simulink model "TXsystem"  (R2024b)
settings: Solver=FixedStepAuto  StartTime=0.0  StopTime=inf  RelTol=1e-3
InitFcn:
  | symbolRate = 1e6;        % 1 MHz symbol rate
  | Ts = 1/symbolRate;       % Sample time per symbol
  | samplesPerSymbol = 8;    % Oversampling factor
  | Fs = symbolRate * samplesPerSymbol;  % 8 MHz sample rate
undefined symbols (not defined in the file or in its folder): ip, QAM, usb
libraries: plutoradiolib x1, commfilt2 x1, commdigbbndam3 x1
settings Model: Creator=J_mas  LastModifiedBy=J_mas

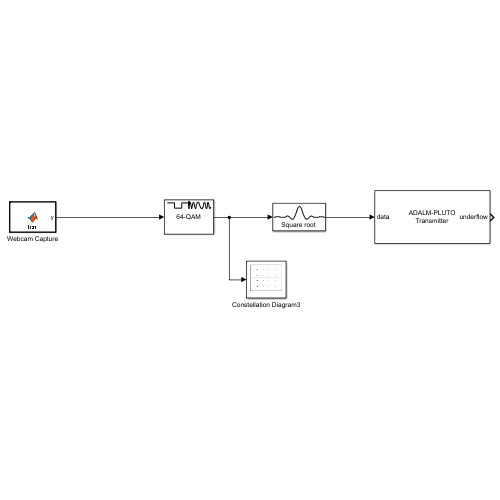
[thumbnail: Simulink's stored preview of the top-level diagram]
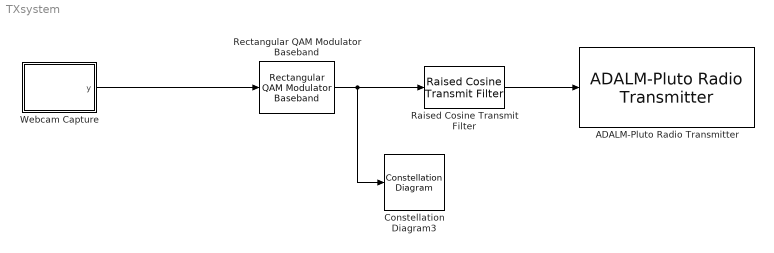
== system TXsystem ==
  ADALM-Pluto Radio Transmitter : plutoradiolib/ADALM-Pluto Radio Transmitter  RadioID=usb:0  uri=ip:10.0.0.200  CenterFrequencySource=Dialog  CenterFrequency=2.4e9  GainSource=Dialog  Gain=-10  ChannelMapping=1  BasebandSampleRate=1e6  UnderflowOutputPort=on  ShowAdvancedProperties=off  UseCustomFilter=off  filtPathRates=[737280000 11520000 3840000 1920000 960000 240000]  filtCoefficients=[-192 82 85 -215 228 -102 -110 290 -318 145 160 -426 471 -215 -238 633 -697 318 349 -923 1009 -457 -498 1309 -1423 640 693 -1812 1959 -876 -945 2458 -2647 1180 1268 -3290 3534 -1572 -1688 4375 -4698 2091 2247 -5836 6284 -2807 -3031 7918 -8588 3870 4225 -11182 12324 -5662 -6330 17255 -19735 9507 11312 -33568 43355 -25227 -42139 305542 305542 -42139 -25227 43355 -33568 11312 9507 -19735 17255 -6330 -5662 12324 -11182 4225 3870 -8588 7918 -3031 -2807 6284 -5836 2247 2091 -4698 4375 -1688 -1572 3534 -3290 1268 1180 -2647 2458 -945 -876 1959 -1812 693 640 -1423 1309 -498 -457 1009 -923 349 318 -697 633 -238 -215 471 -426 160 145 -318 290 -110 -102 228 -215 85 82 -192]  filtCoefficientSize=128  filtDecimInterpFactor=4  filtGain=-12  filtRFBandwidth=18000000  filterConfigStruct=struct()  DataSourceSelect=Input Port  DDSTone1Freq=5e3  DDSTone2Freq=10e3  DDSTone1Scale=0.5  DDSTone2Scale=0.25  DataTimeout=Inf  FrequencyCorrection=0  ENSMPinControlMode=None  BISTLoopbackMode=Disabled  BISTToneInject=Disabled  BISTSignalGen=PRBS  BISTToneFreq=Fs/32  BISTToneLevel=0
  Constellation Diagram3 : ConstellationDiagram  WindowPosition=[504.000000,298.000000,220.000000,313.000000,]  Visible=on  ScopeFrameLocation=window  SamplesPerSymbol=8  SymbolsToDisplaySource=Property  SymbolsToDisplay=100  ReferenceConstellation=64-QAM  XLimits=[-3.19,3.19]  YLimits=[-2.54,2.54]
  Raised Cosine Transmit Filter : commfilt2/Raised Cosine Transmit Filter  filtType=Square root  R=0.2  filtSpan=10  N=8  filterGain=1  InputProcessing=Columns as channels (frame based)  RateOptions=Enforce single-rate processing  framing=Mute  checkCoeff=off  variableName=rcTxFilt  checkGain=Normalized  sampMode=Mute  saveAsFlag=0  currentFiltSpan=10  D=(10)/2  launchFVT=on  roundingMode=Floor  overflowMode=off  coeffDataTypeStr=Inherit: Same word length as input  coeffMin=[]  coeffMax=[]  coeffLastDataTypeStr=Inherit: Same word length as input  outputDataTypeStr=Inherit: Same as accumulator  outputMin=[]  outputMax=[]  outputLastDataTypeStr=Inherit: Same as accumulator
  Rectangular QAM Modulator Baseband : commdigbbndam3/Rectangular QAM Modulator Baseband  M=64  InType=Integer  Enc=Gray  Mapping=[0:15]  PowType=Min. distance between symbols  MinDist=2  AvgPow=1  PeakPow=1  Ph=0  outDtype=double  outWordLen=16  outUDDataType=sfix(16)  outFracLenMode=Best precision  outFracLen=15  outDataTypeStr=double  outLastDataTypeStr=double
  Webcam Capture : MATLAB Function  TreatAsAtomicUnit=on  SystemSampleTime=1/40000
  wires:
  Rectangular QAM Modulator Baseband/1 -> Constellation Diagram3/1, Raised Cosine Transmit Filter/1
  Raised Cosine Transmit Filter/1 -> ADALM-Pluto Radio Transmitter/1
  Webcam Capture/1(y) -> Rectangular QAM Modulator Baseband/1

== matlab function TXsystem/Webcam Capture ==
  data: y output
function y = fcn() %#codegen
    coder.extrinsic('webcam', 'snapshot', 'imresize', 'rgb2gray', 'imshow', 'tic', 'toc', 'fprintf');
    
    persistent cam packetBuffer packetIndex initialized startTime symbolCount
    
    y = uint8(0); % Output type should match Modulator input (usually integer)
    
    % Barker code parameters
    BARKER_LENGTH = 13; % Length-13 Barker code for good autocorrelation
    IMG_ROWS = 100;
    IMG_COLS = 100;
    PAYLOAD_LENGTH = IMG_ROWS * IMG_COLS;

    PACKET_LENGTH = BARKER_LENGTH + PAYLOAD_LENGTH;
    
    if isempty(initialized)
        cam = webcam(1);
        startTime = tic;
        
        % Buffer now holds complete packets (preamble + payload)
        packetBuffer = uint8(zeros(PACKET_LENGTH, 1));
        packetIndex = PACKET_LENGTH + 1; % Start beyond buffer to trigger capture
        symbolCount = 0;
        initialized = true;
    end
    
    % When we've transmitted the entire packet, capture a new frame
    if packetIndex > PACKET_LENGTH
        % Capture and process webcam image
        rawImg = snapshot(cam);
        imgResized = imresize(rawImg, [IMG_ROWS, IMG_COLS]);
        imgGrayRaw = rgb2gray(imgResized);
        %imshow(imgGrayRaw);
        %title('Transmitted Image');
        %drawnow;
        
        
        imgGray = uint8(zeros(IMG_ROWS, IMG_COLS));
        imgGray = imgGrayRaw;
        
        % Flatten the image and convert to 6-bit symbols (0-63)
        temp = reshape(imgGray, PAYLOAD_LENGTH, 1);
        payload = uint8(floor(double(temp) / 4)); % Map 0-255 to 0-63
        
        % Create Barker code preamble
        % Standard 13-bit Barker: [1 1 1 1 1 -1 -1 1 1 -1 1 -1 1]
        % Map to 6-bit symbols: use 63 for '1' and 0 for '-1' for good separation
        barker_preamble = uint8([63 63 63 63 63 0 0 63 63 0 63 0 63]');
        
        % Construct packet: [Preamble | Payload]
        packetBuffer(1:BARKER_LENGTH) = barker_preamble;
        packetBuffer(BARKER_LENGTH+1:PACKET_LENGTH) = payload;
        
        % Reset index to start of packet
        packetIndex = 1;
        
        % Statistics
        elapsedTime = toc(startTime);
        symbolRate = symbolCount / elapsedTime;
        fprintf('Symbol Rate: %.2f symbols/sec\n', symbolRate);
        fprintf('Packet Rate: %.2f frames/sec\n', symbolCount / (PACKET_LENGTH * elapsedTime));
    end
    
    % Output one symbol per call
    if packetIndex <= PACKET_LENGTH
        y = packetBuffer(packetIndex);
        packetIndex = packetIndex + 1;
        symbolCount = symbolCount + 1;
    end
end
